simulink model "Practica4"  (R2020b)
settings: Solver=VariableStepAuto  StartTime=0.0  StopTime=10.0  RelTol=1e-3
undefined symbols (not defined in the file): fv1, fv2, Kr, Kt, Kv, L1, L2, m1, m2, Ra
settings Model: Creator=Danie  LastModifiedBy=Danie

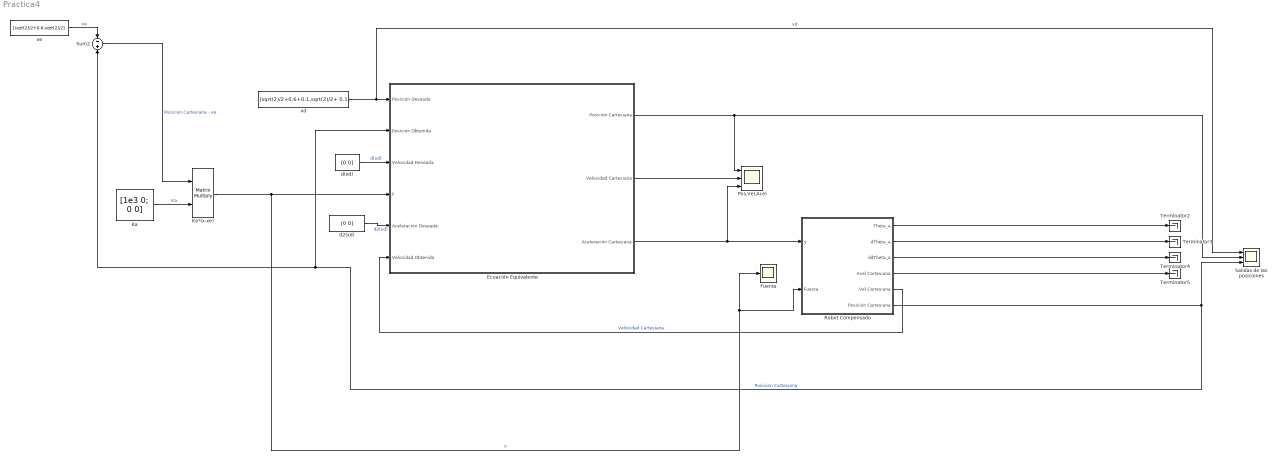
== system Practica4 ==
  Ecuación Equivalente : Subsystem
  "Fuerza " : Scope
  Ka : Constant  Value=[1e3 0; 0 0]
  Ka*(x-xe) : Product  Multiplication=Matrix(*)
  "Pos,Vel,Acel " : Scope  NumInputPorts=3
  Robot Compensado : Subsystem
  Salidas de las posiciones : Scope  NumInputPorts=3
  Sum2 : Sum  Inputs=-+
  Terminator{2..5} (4 alike) : Terminator
  "d(xd) " : Constant  Value=[0 0]
  "d2(xd) " : Constant  Value=[0 0]
  xd : Constant  Value=[sqrt(2)/2+0.6+0.1,sqrt(2)/2+ 0.1]
  xe : Constant  Value=[sqrt(2)/2+0.6,sqrt(2)/2]
  wires:
  "d(xd) "/1 -> Ecuación Equivalente/3("Velocidad Deseada ")  "d(xd)"
  Ka/1 -> Ka*(x-xe)/2  "Ka"
  xd/1 -> Salidas de las posiciones/1, Ecuación Equivalente/1(Posición Deseada)  "xd"
  Robot Compensado/5(Vel Cartesiana) -> Ecuación Equivalente/6("Velocidad Obtenida ")  "Velocidad Cartesiana"
  Robot Compensado/6(Posición Cartesiana) -> Salidas de las posiciones/3, Sum2/2, Ecuación Equivalente/2(Posición Obtenida)  "Posición Cartesiana"
  "d2(xd) "/1 -> Ecuación Equivalente/5(Aceleración Deseada)  "d2(xd)"
  Ecuación Equivalente/3(Aceleración Cartesiana) -> "Pos,Vel,Acel "/3, Robot Compensado/1(y)
  Sum2/1 -> Ka*(x-xe)/1  "Posicion Cartesiana - xe"
  xe/1 -> Sum2/1  "xe"
  Robot Compensado/4(Acel Cartesiana) -> Terminator5/1
  Ka*(x-xe)/1 -> "Fuerza "/1, Robot Compensado/2("Fuerza "), Ecuación Equivalente/4(F)  "F"
  Robot Compensado/3(ddTheta_a) -> Terminator4/1
  Ecuación Equivalente/2(Velocidad Cartesiana) -> "Pos,Vel,Acel "/2
  Robot Compensado/2(dTheta_a) -> Terminator3/1
  Robot Compensado/1("Theta_a ") -> Terminator2/1
  Ecuación Equivalente/1(Posición Cartesiana) -> "Pos,Vel,Acel "/1, Salidas de las posiciones/2

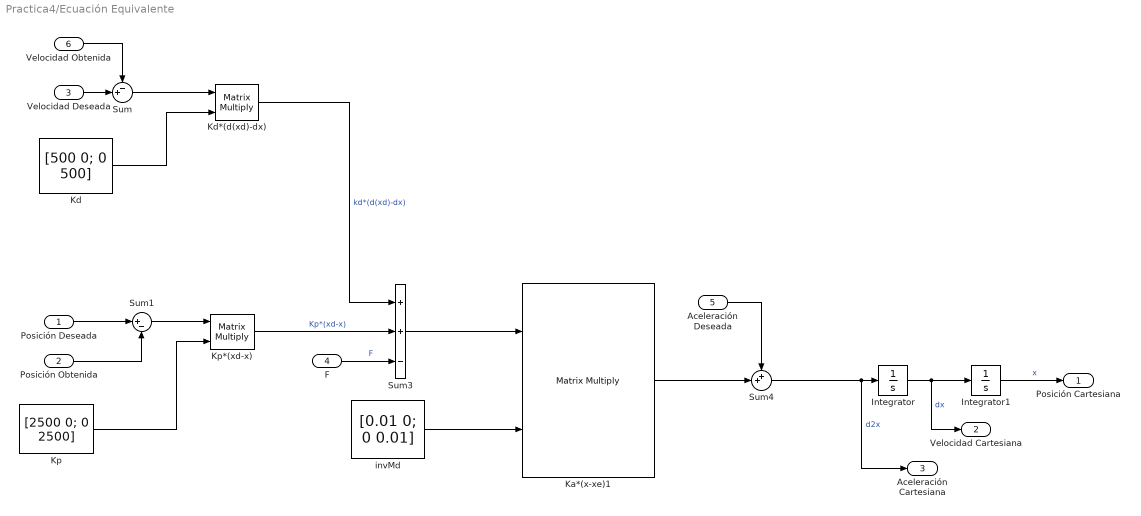
== system Practica4/Ecuación Equivalente ==
  Posición Deseada : Inport
  Posición Obtenida : Inport  Port=2
  "Velocidad Deseada " : Inport  Port=3
  F : Inport  Port=4
  Aceleración Deseada : Inport  Port=5
  "Velocidad Obtenida " : Inport  Port=6
  Integrator : Integrator  ZeroCross=off
  Integrator1 : Integrator  InitialCondition=[sqrt(2)/2+0.6,sqrt(2)/2]
  "Ka*(x-xe)1 " : Product  Multiplication=Matrix(*)
  "Kd " : Constant  Value=[500 0; 0 500]
  "Kd*(d(xd)-dx) " : Product  Multiplication=Matrix(*)
  "Kp " : Constant  Value=[2500 0; 0 2500]
  Kp*(xd-x) : Product  Multiplication=Matrix(*)
  Sum : Sum  Inputs=-+|
  Sum1 : Sum  Inputs=|+-
  Sum3 : Sum  Inputs=++-
  Sum4 : Sum  Inputs=++|
  "invMd " : Constant  Value=[0.01 0; 0 0.01]
  Posición Cartesiana : Outport
  Velocidad Cartesiana : Outport  Port=2
  Aceleración Cartesiana : Outport  Port=3
  wires:
  Kp*(xd-x)/1 -> Sum3/2  "Kp*(xd-x)"
  Sum/1 -> "Kd*(d(xd)-dx) "/1
  Posición Deseada/1 -> Sum1/1
  Sum4/1 -> Integrator/1, Aceleración Cartesiana/1  "d2x"
  "Velocidad Obtenida "/1 -> Sum/1
  Integrator1/1 -> Posición Cartesiana/1  "x"
  Aceleración Deseada/1 -> Sum4/1
  Sum3/1 -> "Ka*(x-xe)1 "/1
  "Kd "/1 -> "Kd*(d(xd)-dx) "/2
  "Ka*(x-xe)1 "/1 -> Sum4/2
  "Kd*(d(xd)-dx) "/1 -> Sum3/1  "kd*(d(xd)-dx)"
  Sum1/1 -> Kp*(xd-x)/1
  Integrator/1 -> Integrator1/1, Velocidad Cartesiana/1  "dx"
  "invMd "/1 -> "Ka*(x-xe)1 "/2
  "Kp "/1 -> Kp*(xd-x)/2
  "Velocidad Deseada "/1 -> Sum/2
  Posición Obtenida/1 -> Sum1/2
  F/1 -> Sum3/3  "F"

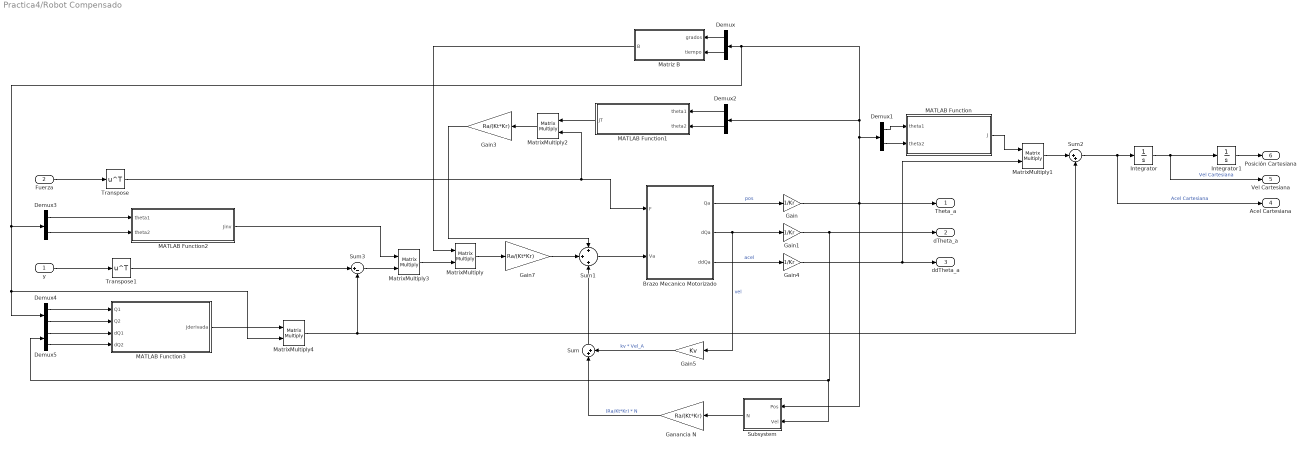
== system Practica4/Robot Compensado ==
  y : Inport
  "Fuerza " : Inport  Port=2
  Brazo Mecanico Motorizado : Subsystem  mask{Ra=0.3, kt=0.5, kv=0.5, Kr1=100, Kr2=100, sat_rpm=1500}
      mask prompts: Ra "Resistencia de la armadura del motor (Ra)"; kt "Constante de conversiòn de tensiòn-par (kt)"; kv "Constante de la fuerzaq contra-electromotriz (kv)"; Kr1 "Reductor del actuador 1 (Kr1)"; Kr2 "Reductor del actuador 2 (Kr2)"; sat_rpm "rpm max actuadores"
  Demux{,1..5} (6 alike) : Demux  Outputs=2
  Gain : Gain  Gain=1/Kr
  Gain1 : Gain  Gain=1/Kr
  Gain3 : Gain  Gain=Ra/(Kt*Kr)
  Gain4 : Gain  Gain=1/Kr
  Gain5 : Gain  Gain=Kv
  Gain7 : Gain  Gain=Ra/(Kt*Kr)
  "Ganancia N " : Gain  Gain=Ra/(Kt*Kr)
  Integrator : Integrator
  Integrator1 : Integrator  InitialCondition=[sqrt(2)/2+0.6,sqrt(2)/2]
  MATLAB Function : MATLAB Function  TreatAsAtomicUnit=on
  MATLAB Function1 : MATLAB Function  TreatAsAtomicUnit=on
  MATLAB Function2 : MATLAB Function  TreatAsAtomicUnit=on
  MATLAB Function3 : MATLAB Function  TreatAsAtomicUnit=on
  MatrixMultiply{,1..4} (5 alike) : Product  Multiplication=Matrix(*)
  Matriz B : MATLAB Function  TreatAsAtomicUnit=on
  Subsystem : Subsystem
  Sum : Sum  Inputs=|++
  Sum1 : Sum  Inputs=+|+|+
  Sum2 : Sum  Inputs=|++
  Sum3 : Sum  Inputs=|+-
  Transpose : Math  Operator=transpose  SaturateOnIntegerOverflow=on
  Transpose1 : Math  Operator=transpose  SaturateOnIntegerOverflow=on
  "Theta_a " : Outport
  dTheta_a : Outport  Port=2
  ddTheta_a : Outport  Port=3
  Acel Cartesiana : Outport  Port=4
  Vel Cartesiana : Outport  Port=5
  Posición Cartesiana : Outport  Port=6
  wires:
  Demux/1 -> Matriz B/1(grados)
  Brazo Mecanico Motorizado/3(ddQa) -> Gain4/1  "acel"
  Subsystem/1("N ") -> "Ganancia N "/1
  Demux/2 -> Matriz B/2(tiempo)
  "Ganancia N "/1 -> Sum/1  "(Ra/Kt*Kr) * N"
  Gain5/1 -> Sum/2  "kv * Vel_A"
  Sum/1 -> Sum1/3
  Brazo Mecanico Motorizado/2(dQa) -> Gain5/1, Gain1/1  "vel"
  Gain7/1 -> Sum1/2
  Brazo Mecanico Motorizado/1(Qa) -> Gain/1  "pos"
  Demux1/1 -> MATLAB Function/1(theta1)
  Demux1/2 -> MATLAB Function/2(theta2)
  MATLAB Function/1(J) -> MatrixMultiply1/1
  Gain4/1 -> ddTheta_a/1, MatrixMultiply1/2
  MatrixMultiply1/1 -> Sum2/1
  Sum2/1 -> Acel Cartesiana/1, Integrator/1  "Acel Cartesiana"
  Integrator/1 -> Integrator1/1, Vel Cartesiana/1  "Vel Cartesiana"
  Integrator1/1 -> Posición Cartesiana/1
  Demux2/2 -> MATLAB Function1/2(theta2)
  Demux2/1 -> MATLAB Function1/1(theta1)
  MATLAB Function1/1(JT) -> MatrixMultiply2/1
  MatrixMultiply2/1 -> Gain3/1
  Demux3/1 -> MATLAB Function2/1(theta1)
  Demux3/2 -> MATLAB Function2/2(theta2)
  Transpose1/1 -> Sum3/1
  MatrixMultiply3/1 -> MatrixMultiply/2
  MATLAB Function2/1(Jinv) -> MatrixMultiply3/1
  MATLAB Function3/1(Jderivada) -> MatrixMultiply4/1
  MatrixMultiply4/1 -> Sum3/2, Sum2/2
  Sum1/1 -> Brazo Mecanico Motorizado/2(Va)
  Demux4/1 -> MATLAB Function3/1(Q1)
  Demux4/2 -> MATLAB Function3/2(Q2)
  Gain/1 -> Subsystem/1(Pos), "Theta_a "/1, Demux1/1, Demux4/1, MatrixMultiply4/2, Demux3/1, Demux/1, Demux2/1
  Demux5/2 -> MATLAB Function3/4(dQ2)
  Demux5/1 -> MATLAB Function3/3(dQ1)
  Gain1/1 -> Demux5/1, Subsystem/2(Vel), dTheta_a/1
  Sum3/1 -> MatrixMultiply3/2
  Transpose/1 -> Brazo Mecanico Motorizado/1(F), MatrixMultiply2/2
  MatrixMultiply/1 -> Gain7/1
  "Fuerza "/1 -> Transpose/1
  y/1 -> Transpose1/1
  Gain3/1 -> Sum1/1
  Matriz B/1(B) -> MatrixMultiply/1

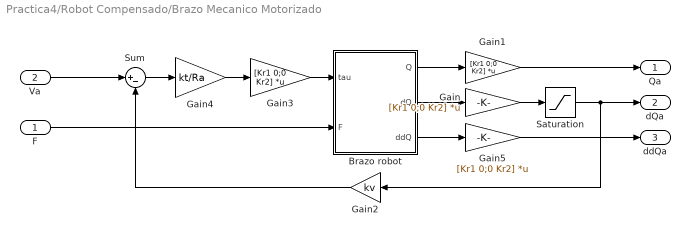
== system Practica4/Robot Compensado/Brazo Mecanico Motorizado ==
  F : Inport
  Va : Inport  Port=2
  Brazo robot : Subsystem  mask{m1=10, m2=4, L1=1, L2=0.6, fv1=2.5, fv2=1.5}
      mask prompts: m1 "Masa 1"; m2 "Masa 2"; L1 "Longitud 1"; L2 "Longitud 2"; fv1 "Friccion 1"; fv2 "Friccion 2"
  Gain{,1,3,5} (4 alike) : Gain  Gain=[Kr1 0;0 Kr2]  Multiplication=Matrix(K*u) (u vector)
  Gain2 : Gain  Gain=kv
  Gain4 : Gain  Gain=kt/Ra
  Saturation : Saturate  UpperLimit=sat_rpm*2*pi/60  LowerLimit=-sat_rpm*2*pi/60
  Sum : Sum  Inputs=|+-
  Qa : Outport
  dQa : Outport  Port=2
  ddQa : Outport  Port=3
  wires:
  Brazo robot/1(Q) -> Gain1/1
  Brazo robot/2(dQ) -> Gain/1
  Gain/1 -> Saturation/1
  Gain2/1 -> Sum/2
  Sum/1 -> Gain4/1
  Gain4/1 -> Gain3/1
  Gain3/1 -> Brazo robot/1(tau)
  Gain1/1 -> Qa/1
  Saturation/1 -> Gain2/1, dQa/1
  Brazo robot/3(ddQ) -> Gain5/1
  Gain5/1 -> ddQa/1
  F/1 -> Brazo robot/2(F)
  Va/1 -> Sum/1

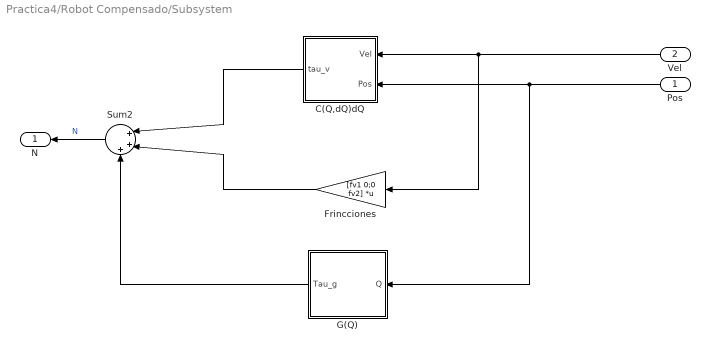
== system Practica4/Robot Compensado/Subsystem ==
  Pos : Inport
  Vel : Inport  Port=2
  C(Q,dQ)dQ : Subsystem
  Frincciones : Gain  Gain=[fv1 0;0 fv2]  Multiplication=Matrix(K*u)  SaturateOnIntegerOverflow=on  OutDataTypeStr=Inherit: Same as input  ParamDataTypeStr=Inherit: Same as input
  G(Q) : Subsystem
  Sum2 : Sum  Inputs=|+++
  "N " : Outport
  wires:
  Frincciones/1 -> Sum2/2
  G(Q)/1(Tau_g) -> Sum2/3
  Vel/1 -> C(Q,dQ)dQ/1(Vel), Frincciones/1
  C(Q,dQ)dQ/1(tau_v) -> Sum2/1
  Sum2/1 -> "N "/1  "N"
  Pos/1 -> G(Q)/1(Q), C(Q,dQ)dQ/2("Pos ")

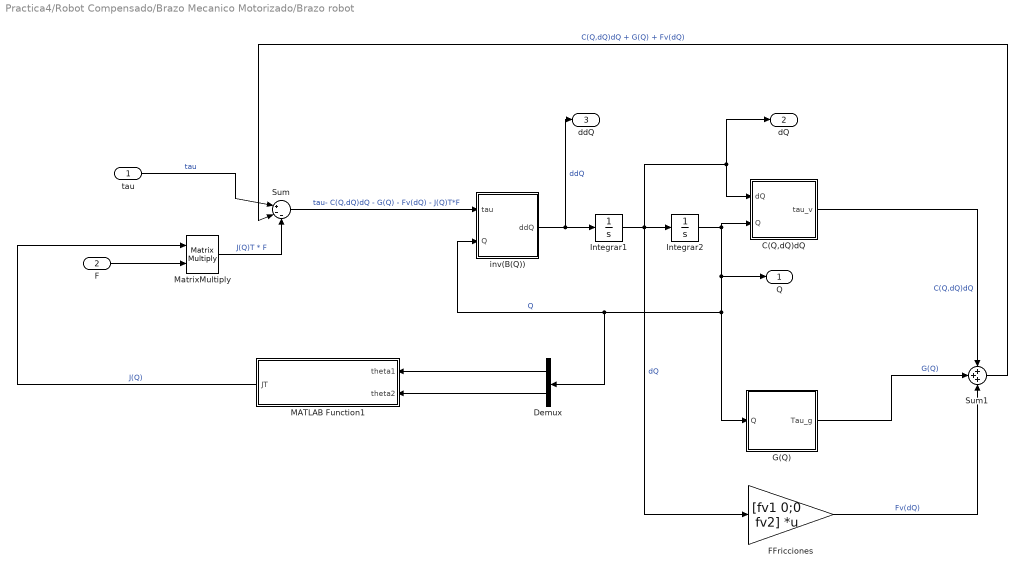
== system Practica4/Robot Compensado/Brazo Mecanico Motorizado/Brazo robot ==
  tau : Inport
  F : Inport  Port=2
  C(Q,dQ)dQ : Subsystem
  Demux : Demux  Outputs=2
  FFricciones : Gain  Gain=[fv1 0;0 fv2]  Multiplication=Matrix(K*u)  SaturateOnIntegerOverflow=on  OutDataTypeStr=Inherit: Same as input  ParamDataTypeStr=Inherit: Same as input
  G(Q) : Subsystem
  Integrar1 : Integrator  InitialCondition=[0,0]
  Integrar2 : Integrator  InitialCondition=[45*pi/180,-45*pi/180]
  MATLAB Function1 : MATLAB Function  TreatAsAtomicUnit=on
  MatrixMultiply : Product  Multiplication=Matrix(*)
  Sum : Sum  Inputs=|+--  SaturateOnIntegerOverflow=on
  Sum1 : Sum  Inputs=+++  SaturateOnIntegerOverflow=on
  inv(B(Q)) : Subsystem
  Q : Outport
  dQ : Outport  Port=2
  ddQ : Outport  Port=3
  wires:
  tau/1 -> Sum/1  "tau"
  Sum/1 -> inv(B(Q))/1(tau)  "tau- C(Q,dQ)dQ - G(Q) - Fv(dQ) - J(Q)T*F"
  inv(B(Q))/1(ddQ) -> Integrar1/1, ddQ/1  "ddQ"
  Integrar1/1 -> dQ/1, C(Q,dQ)dQ/1(dQ), Integrar2/1, FFricciones/1  "dQ"
  Integrar2/1 -> Q/1, inv(B(Q))/2(Q), Demux/1, G(Q)/1(Q), C(Q,dQ)dQ/2(Q)  "Q"
  C(Q,dQ)dQ/1(tau_v) -> Sum1/1  "C(Q,dQ)dQ"
  G(Q)/1(Tau_g) -> Sum1/2  "G(Q)"
  Sum1/1 -> Sum/2  "C(Q,dQ)dQ + G(Q) + Fv(dQ)"
  FFricciones/1 -> Sum1/3  "Fv(dQ)"
  Demux/1 -> MATLAB Function1/1(theta1)
  Demux/2 -> MATLAB Function1/2(theta2)
  MatrixMultiply/1 -> Sum/3  "J(Q)T * F"
  MATLAB Function1/1(JT) -> MatrixMultiply/1  "J(Q)"
  F/1 -> MatrixMultiply/2

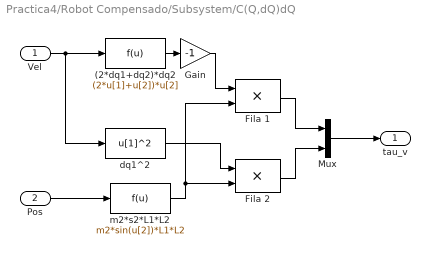
== system Practica4/Robot Compensado/Subsystem/C(Q,dQ)dQ ==
  Vel : Inport
  "Pos " : Inport  Port=2
  (2*dq1+dq2)*dq2 : Fcn  Expr=(2*u[1]+u[2])*u[2]
  Fila 1 : Product  SaturateOnIntegerOverflow=on  OutDataTypeStr=Inherit: Same as first input
  Fila 2 : Product  SaturateOnIntegerOverflow=on  OutDataTypeStr=Inherit: Same as first input
  Gain : Gain  Gain=-1  SaturateOnIntegerOverflow=on  OutDataTypeStr=Inherit: Same as input  ParamDataTypeStr=Inherit: Same as input
  Mux : Mux  Inputs=2
  dq1^2 : Fcn  Expr=u[1]^2
  m2*s2*L1*L2 : Fcn  Expr=m2*sin(u[2])*L1*L2
  tau_v : Outport
  wires:
  "Pos "/1 -> m2*s2*L1*L2/1
  m2*s2*L1*L2/1 -> Fila 2/2, Fila 1/2
  Vel/1 -> (2*dq1+dq2)*dq2/1, dq1^2/1
  dq1^2/1 -> Fila 2/1
  Fila 1/1 -> Mux/1
  Fila 2/1 -> Mux/2
  Mux/1 -> tau_v/1
  (2*dq1+dq2)*dq2/1 -> Gain/1
  Gain/1 -> Fila 1/1

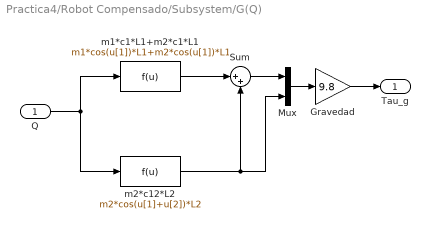
== system Practica4/Robot Compensado/Subsystem/G(Q) ==
  Q : Inport
  Gravedad : Gain  Gain=9.8  SaturateOnIntegerOverflow=on  OutDataTypeStr=Inherit: Same as input  ParamDataTypeStr=Inherit: Same as input
  Mux : Mux  Inputs=2
  Sum : Sum  Inputs=|++  SaturateOnIntegerOverflow=on
  m1*c1*L1+m2*c1*L1 : Fcn  Expr=m1*cos(u[1])*L1+m2*cos(u[1])*L1
  m2*c12*L2 : Fcn  Expr=m2*cos(u[1]+u[2])*L2
  Tau_g : Outport
  wires:
  m1*c1*L1+m2*c1*L1/1 -> Sum/1
  m2*c12*L2/1 -> Sum/2, Mux/2
  Sum/1 -> Mux/1
  Q/1 -> m1*c1*L1+m2*c1*L1/1, m2*c12*L2/1
  Gravedad/1 -> Tau_g/1
  Mux/1 -> Gravedad/1

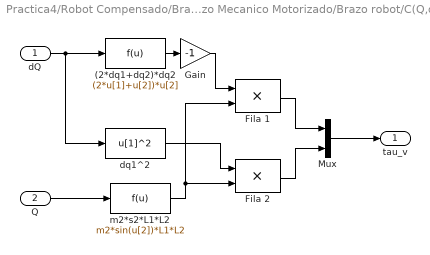
== system Practica4/Robot Compensado/Brazo Mecanico Motorizado/Brazo robot/C(Q,dQ)dQ ==
  dQ : Inport
  Q : Inport  Port=2
  (2*dq1+dq2)*dq2 : Fcn  Expr=(2*u[1]+u[2])*u[2]
  Fila 1 : Product  SaturateOnIntegerOverflow=on  OutDataTypeStr=Inherit: Same as first input
  Fila 2 : Product  SaturateOnIntegerOverflow=on  OutDataTypeStr=Inherit: Same as first input
  Gain : Gain  Gain=-1  SaturateOnIntegerOverflow=on  OutDataTypeStr=Inherit: Same as input  ParamDataTypeStr=Inherit: Same as input
  Mux : Mux  Inputs=2
  dq1^2 : Fcn  Expr=u[1]^2
  m2*s2*L1*L2 : Fcn  Expr=m2*sin(u[2])*L1*L2
  tau_v : Outport
  wires:
  Q/1 -> m2*s2*L1*L2/1
  m2*s2*L1*L2/1 -> Fila 2/2, Fila 1/2
  dQ/1 -> (2*dq1+dq2)*dq2/1, dq1^2/1
  dq1^2/1 -> Fila 2/1
  Fila 1/1 -> Mux/1
  Fila 2/1 -> Mux/2
  Mux/1 -> tau_v/1
  (2*dq1+dq2)*dq2/1 -> Gain/1
  Gain/1 -> Fila 1/1

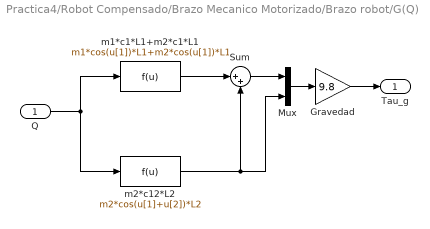
== system Practica4/Robot Compensado/Brazo Mecanico Motorizado/Brazo robot/G(Q) ==
  Q : Inport
  Gravedad : Gain  Gain=9.8  SaturateOnIntegerOverflow=on  OutDataTypeStr=Inherit: Same as input  ParamDataTypeStr=Inherit: Same as input
  Mux : Mux  Inputs=2
  Sum : Sum  Inputs=|++  SaturateOnIntegerOverflow=on
  m1*c1*L1+m2*c1*L1 : Fcn  Expr=m1*cos(u[1])*L1+m2*cos(u[1])*L1
  m2*c12*L2 : Fcn  Expr=m2*cos(u[1]+u[2])*L2
  Tau_g : Outport
  wires:
  m1*c1*L1+m2*c1*L1/1 -> Sum/1
  m2*c12*L2/1 -> Sum/2, Mux/2
  Sum/1 -> Mux/1
  Q/1 -> m1*c1*L1+m2*c1*L1/1, m2*c12*L2/1
  Gravedad/1 -> Tau_g/1
  Mux/1 -> Gravedad/1

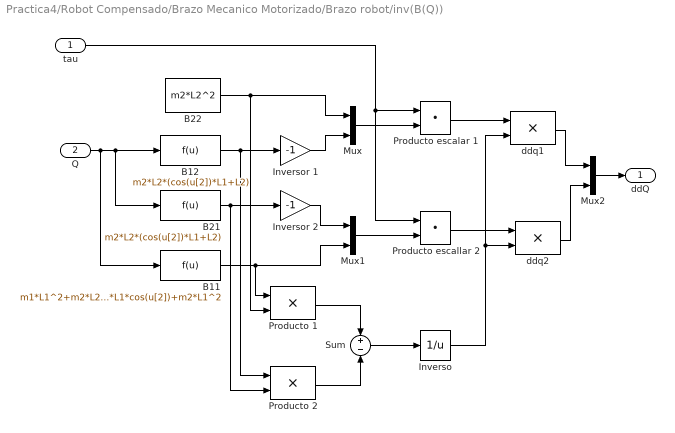
== system Practica4/Robot Compensado/Brazo Mecanico Motorizado/Brazo robot/inv(B(Q)) ==
  tau : Inport
  Q : Inport  Port=2
  B11 : Fcn  Expr=m1*L1^2+m2*L2^2+2*m2*L2*L1*cos(u[2])+m2*L1^2
  B12 : Fcn  Expr=m2*L2*(cos(u[2])*L1+L2)
  B21 : Fcn  Expr=m2*L2*(cos(u[2])*L1+L2)
  B22 : Constant  Value=m2*L2^2
  Inverso : Math  Operator=reciprocal  SignedPower=on  SaturateOnIntegerOverflow=on
  Inversor 1 : Gain  Gain=-1  SaturateOnIntegerOverflow=on  OutDataTypeStr=Inherit: Same as input  ParamDataTypeStr=Inherit: Same as input
  Inversor 2 : Gain  Gain=-1  SaturateOnIntegerOverflow=on  OutDataTypeStr=Inherit: Same as input  ParamDataTypeStr=Inherit: Same as input
  Mux : Mux  Inputs=2
  Mux1 : Mux  Inputs=2
  Mux2 : Mux  Inputs=2
  Producto 1 : Product  SaturateOnIntegerOverflow=on  OutDataTypeStr=Inherit: Same as first input
  Producto 2 : Product  SaturateOnIntegerOverflow=on  OutDataTypeStr=Inherit: Same as first input
  Producto escalar 1 : DotProduct  InputSameDT=on  OutDataTypeStr=Inherit: Inherit via internal rule
  Producto escallar 2 : DotProduct  InputSameDT=on  OutDataTypeStr=Inherit: Inherit via internal rule
  Sum : Sum  Inputs=+-  SaturateOnIntegerOverflow=on
  ddq1 : Product  SaturateOnIntegerOverflow=on  OutDataTypeStr=Inherit: Same as first input
  ddq2 : Product  SaturateOnIntegerOverflow=on  OutDataTypeStr=Inherit: Same as first input
  ddQ : Outport
  wires:
  Q/1 -> B12/1, B21/1, B11/1
  B12/1 -> Inversor 1/1, Producto 2/1
  B21/1 -> Inversor 2/1, Producto 2/2
  B22/1 -> Mux/1, Producto 1/2
  Inversor 1/1 -> Mux/2
  Inversor 2/1 -> Mux1/1
  B11/1 -> Mux1/2, Producto 1/1
  Mux/1 -> Producto escalar 1/2
  tau/1 -> Producto escalar 1/1, Producto escallar 2/1
  Mux1/1 -> Producto escallar 2/2
  Producto 1/1 -> Sum/1
  Producto 2/1 -> Sum/2
  Sum/1 -> Inverso/1
  Producto escalar 1/1 -> ddq1/1
  Producto escallar 2/1 -> ddq2/1
  Inverso/1 -> ddq1/2, ddq2/2
  ddq1/1 -> Mux2/1
  ddq2/1 -> Mux2/2
  Mux2/1 -> ddQ/1

== matlab function Practica4/Robot Compensado/MATLAB Function ==
  data: theta1 input; J output; theta2 input
function J = JacobianaSalida(theta1,theta2)
L1 = 1;
L2 = 0.6;
a = -L1*sin(theta1)-L2*sin(theta1+theta2);
b = -L2*sin(theta1+theta2);
c = L1*cos(theta1)+L2*cos(theta1+theta2);
d = L2*cos(theta1+theta2);

J = [a b; c d];

== matlab function Practica4/Robot Compensado/Matriz B ==
  data: grados input; B output; tiempo input
function B = MatrizB(grados,tiempo)

m1 =10;
m2 = 4;
L1 = 1;
L2 = 0.6;
fr1 = 2.5;
fr2 = 1.5;


B11 = m1*L1^2 + m2*L2^2 + 2*m2*L2*L1*cos(tiempo) + m2*L1^2; 
B12 = m2*L2*(cos(tiempo)*L1+L2);
B21 = m2*L2*(cos(tiempo)*L1+L2);
B22 = m2*L2^2;

B = [B11, B12; B21, B22];

== matlab function Practica4/Robot Compensado/MATLAB Function1 ==
  data: theta1 input; JT output; theta2 input
function JT = JacobianaT(theta1,theta2)
L1 = 1;
L2 = 0.6;
a = -L1*sin(theta1)-L2*sin(theta1+theta2);
b = -L2*sin(theta1+theta2);
c = L1*cos(theta1)+L2*cos(theta1+theta2);
d = L2*cos(theta1+theta2);

JT = [a b; c d]';

== matlab function Practica4/Robot Compensado/MATLAB Function2 ==
  data: theta1 input; Jinv output; theta2 input
function Jinv = JacobianaInversa(theta1,theta2)
L1 = 1;
L2 = 0.6;
a = -L1*sin(theta1)-L2*sin(theta1+theta2);
b = -L2*sin(theta1+theta2);
c = L1*cos(theta1)+L2*cos(theta1+theta2);
d = L2*cos(theta1+theta2);

J = [a b; c d];
Jinv = inv(J);

== matlab function Practica4/Robot Compensado/MATLAB Function3 ==
  data: Q1 input; Jderivada output; Q2 input; dQ1 input; dQ2 input
function Jderivada = DerivadaJacobiana(Q1,Q2,dQ1,dQ2)
L1 = 1;
L2 = 0.6;
a = -L1*cos(Q1)*dQ1-L2*cos(Q1+Q2)*(dQ1+dQ2);
b = -L2*cos(Q1+Q2)*(dQ1+dQ2);
c = -L1*sin(Q1)*dQ1-L2*sin(Q1+Q2)*(dQ1+dQ2);
d = -L2*sin(Q1+Q2)*(dQ1+dQ2);

Jderivada = [a b; c d];

== matlab function Practica4/Robot Compensado/Brazo Mecanico Motorizado/Brazo robot/MATLAB Function1 ==
  data: theta1 input; JT output; theta2 input
function JT = JacobianaT(theta1,theta2)
L1 = 1;
L2 = 0.6;
a = -L1*sin(theta1)-L2*sin(theta1+theta2);
b = -L2*sin(theta1+theta2);
c = L1*cos(theta1)+L2*cos(theta1+theta2);
d = L2*cos(theta1+theta2);

JT = [a b; c d]';
